simulink model "OpenLoopWindTurbineModelTrim2015a"  (R2015a)
settings: Solver=ode4  SolverMode=SingleTasking  StartTime=0.0  StopTime=TIME_SIM  FixedStep=STEP_SIZE  MaxStep=Ts  RelTol=1e-6
undefined symbols (not defined in the file): A, Bd, beta_OP, CP0, Jg, Jr, Kd, Lambda0, Ng, Pitch0, R, rho_air, Tg_OP, v_OP, x0
settings Model: Creator=roga  LastModifiedBy=Fabio Spagnolo
settings DataIOCC: SaveFinalState=on
settings DebuggingCC: UnderspecifiedInitializationDetection=Classic  MergeDetectMultiDrivingBlocksExec=none  SolverPrmCheckMsg=warning  StateNameClashWarn=warning

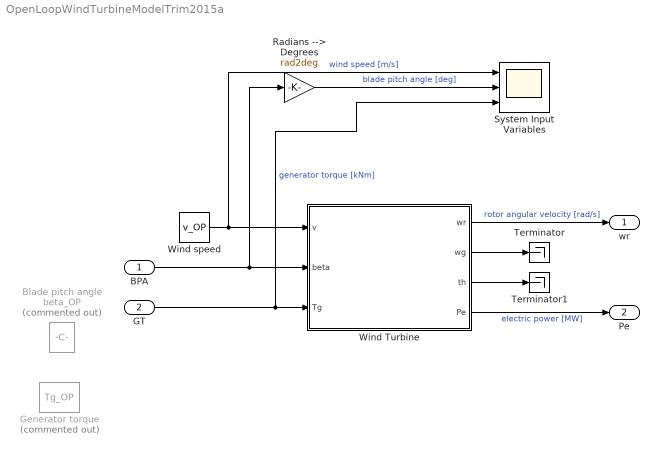
== system OpenLoopWindTurbineModelTrim2015a ==
  BPA : Inport
  GT : Inport  Port=2
  Blade pitch angle : Constant  Commented=on  Value=beta_OP
      mask Display: port_label('output',1,'\beta_{OP}','Interpreter','tex')
  Generator torque : Constant  Commented=on  Value=Tg_OP
      mask Display: port_label('output',1,'T_{g,OP}','Interpreter','tex')
  Radians --> Degrees : Gain  Gain=rad2deg
  System Input Variables : Scope  NumInputPorts=3
      settings: TimeRange=auto  ShowLegends=on  MaxDataPoints=5000  SaveToWorkspace=off  SaveName=ScopeData  YMin=-5~-5~-5  YMax=5~5~5  SampleTime=-1
  Terminator : Terminator
  Terminator1 : Terminator
  Wind Turbine : Subsystem
      mask Display:
      | image('wind_turbine.jpg')
      | port_label('input',1,'v')
      | port_label('input',2,'\beta','Interpreter','tex')
      | port_label('input',3,'T_g','Interpreter','tex')
      | port_label('output',1,'\omega_r','Interpreter','tex')
      | port_label('output',2,'\omega_g','Interpreter','tex')
      | port_label('output',3,'\theta','Interpreter','tex')
      | port_label('output',4,'P_e','Interpreter','tex')
  Wind speed : Constant  Value=v_OP
      mask Display: port_label('output',1,'v_{OP}','Interpreter','tex')
  wr : Outport
  Pe : Outport  Port=2
  wires:
  Wind speed/1 -> Wind Turbine/1(v), System Input Variables/1  "wind speed [m/s]"
  BPA/1 -> Wind Turbine/2(beta), Radians --> Degrees/1
  GT/1 -> Wind Turbine/3(Tg), System Input Variables/3  "generator torque [kNm]"
  Wind Turbine/1(wr) -> wr/1  "rotor angular velocity [rad/s]"
  Wind Turbine/4(Pe) -> Pe/1  "electric power [MW]"
  Radians --> Degrees/1 -> System Input Variables/2  "blade pitch angle [deg]"
  Wind Turbine/3(th) -> Terminator1/1
  Wind Turbine/2(wg) -> Terminator/1

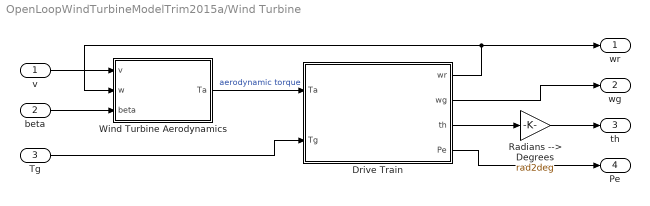
== system OpenLoopWindTurbineModelTrim2015a/Wind Turbine ==
  v : Inport
  beta : Inport  Port=2
  Tg : Inport  Port=3
  Drive Train : Subsystem
      mask Display:
      | image('wind_turbine_nacelle.jpg')
      | port_label('input',1,'T_a','Interpreter','tex')
      | port_label('input',2,'T_g','Interpreter','tex')
      | port_label('output',1,'\omega_r','Interpreter','tex')
      | port_label('output',2,'\omega_g','Interpreter','tex')
      | port_label('output',3,'\theta','Interpreter','tex')
      | port_label('output',4,'P_e','Interpreter','tex')
  Radians --> Degrees : Gain  Gain=rad2deg
  Wind Turbine Aerodynamics : Subsystem
      mask Display:
      | image('PowerCoefficient.jpg')
      | port_label('input',1,'v')
      | port_label('input',2,'\omega_r','Interpreter','tex')
      | port_label('input',3,'\beta','Interpreter','tex')
      | port_label('output',1,'T_a','Interpreter','tex')
  wr : Outport
  wg : Outport  Port=2
  th : Outport  Port=3
  Pe : Outport  Port=4
  wires:
  Drive Train/1(wr) -> wr/1, Wind Turbine Aerodynamics/2(w)
  Tg/1 -> Drive Train/2(Tg)
  Drive Train/2(wg) -> wg/1
  Drive Train/3(th) -> Radians --> Degrees/1
  Drive Train/4(Pe) -> Pe/1
  beta/1 -> Wind Turbine Aerodynamics/3(beta)
  Wind Turbine Aerodynamics/1(Ta) -> Drive Train/1(Ta)  "aerodynamic torque"
  v/1 -> Wind Turbine Aerodynamics/1(v)
  Radians --> Degrees/1 -> th/1

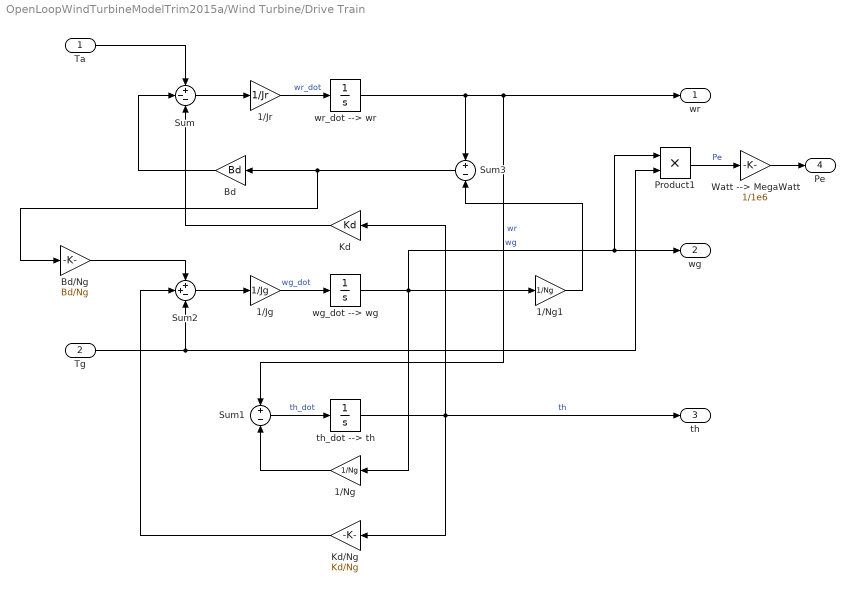
== system OpenLoopWindTurbineModelTrim2015a/Wind Turbine/Drive Train ==
  Ta : Inport
  Tg : Inport  Port=2
  1/Jg : Gain  Gain=1/Jg
  1/Jr : Gain  Gain=1/Jr
  1/Ng : Gain  Gain=1/Ng
  1/Ng1 : Gain  Gain=1/Ng
  Bd : Gain  Gain=Bd
  Bd/Ng : Gain  Gain=Bd/Ng
  Kd : Gain  Gain=Kd
  Kd/Ng : Gain  Gain=Kd/Ng
  Product1 : Product
  Sum : Sum  Inputs=+--
  Sum1 : Sum  Inputs=+-
  Sum2 : Sum  Inputs=++-
  Sum3 : Sum  Inputs=+-
  Watt --> MegaWatt : Gain  Gain=1/1e6
  th_dot --> th : Integrator  Priority=3  InitialCondition=x0(3)  LowerSaturationLimit=0
  wg_dot --> wg : Integrator  Priority=2  InitialCondition=x0(2)  LowerSaturationLimit=0
  wr_dot --> wr : Integrator  Priority=1  InitialCondition=x0(1)  LowerSaturationLimit=0
  wr : Outport
  wg : Outport  Port=2
  th : Outport  Port=3
  Pe : Outport  Port=4
  wires:
  wg_dot --> wg/1 -> Product1/1, wg/1, 1/Ng1/1, 1/Ng/1  "wg"
  wr_dot --> wr/1 -> Sum3/1, wr/1, Sum1/1  "wr"
  1/Ng/1 -> Sum1/2
  Sum1/1 -> th_dot --> th/1  "th_dot"
  Sum2/1 -> 1/Jg/1
  1/Ng1/1 -> Sum3/2
  Sum/1 -> 1/Jr/1
  1/Jr/1 -> wr_dot --> wr/1  "wr_dot"
  th_dot --> th/1 -> th/1, Kd/Ng/1, Kd/1  "th"
  1/Jg/1 -> wg_dot --> wg/1  "wg_dot"
  Sum3/1 -> Bd/Ng/1, Bd/1
  Bd/1 -> Sum/2
  Kd/1 -> Sum/3
  Bd/Ng/1 -> Sum2/1
  Kd/Ng/1 -> Sum2/2
  Ta/1 -> Sum/1
  Tg/1 -> Product1/2, Sum2/3
  Product1/1 -> Watt --> MegaWatt/1  "Pe"
  Watt --> MegaWatt/1 -> Pe/1

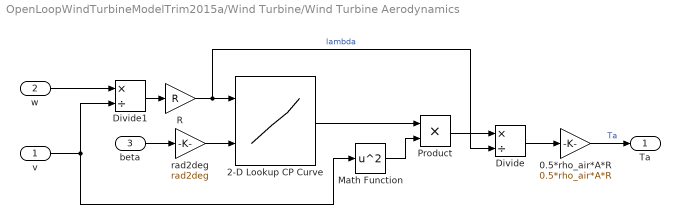
== system OpenLoopWindTurbineModelTrim2015a/Wind Turbine/Wind Turbine Aerodynamics ==
  v : Inport
  w : Inport  Port=2
  beta : Inport  Port=3
  0.5*rho_air*A*R : Gain  Gain=0.5*rho_air*A*R
  2-D Lookup CP Curve : Lookup_n-D  BreakpointsForDimension1=Lambda0  BreakpointsForDimension2=Pitch0  BreakpointsForDimension3=CP0'  Table=CP0  DiagnosticForOutOfRangeInput=Warning  RndMeth=Simplest  InputSameDT=on
  Divide : Product  Inputs=*/
  Divide1 : Product  Inputs=*/
  Math Function : Math  Operator=square  SaturateOnIntegerOverflow=on
  Product : Product
  R : Gain  Gain=R
  rad2deg : Gain  Gain=rad2deg
  Ta : Outport
  wires:
  0.5*rho_air*A*R/1 -> Ta/1  "Ta"
  beta/1 -> rad2deg/1
  w/1 -> Divide1/1
  Divide/1 -> 0.5*rho_air*A*R/1
  Product/1 -> Divide/1
  Math Function/1 -> Product/2
  2-D Lookup CP Curve/1 -> Product/1
  v/1 -> Divide1/2, Math Function/1
  Divide1/1 -> R/1
  R/1 -> Divide/2, 2-D Lookup CP Curve/1  "lambda"
  rad2deg/1 -> 2-D Lookup CP Curve/2
